simulink model "Sim7"  (R2014a)
settings: Solver=ode45  StartTime=0.0  StopTime=10.0  RelTol=1e-3
settings Model: Creator=OCAC  LastModifiedBy=OCAC

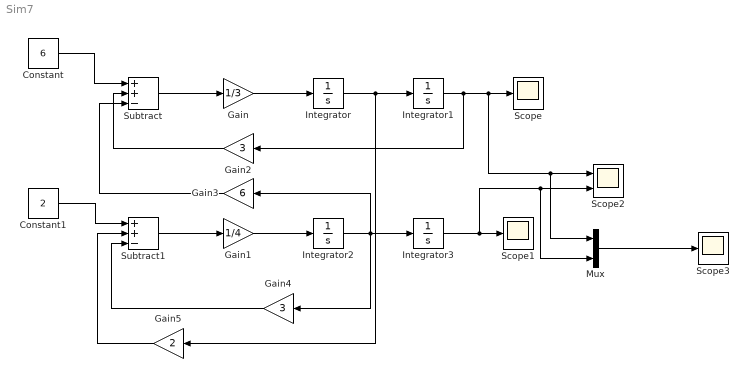
== system Sim7 ==
  Constant : Constant  Value=6
  Constant1 : Constant  Value=2
  Gain : Gain  Gain=1/3
  Gain1 : Gain  Gain=1/4
  Gain2 : Gain  Gain=3
  Gain3 : Gain  Gain=6
  Gain4 : Gain  Gain=3
  Gain5 : Gain  Gain=2
  Integrator{,1..3} (4 alike) : Integrator
  Mux : Mux  Inputs=2
  Scope : Scope
  Scope1 : Scope
  Scope2 : Scope  NumInputPorts=2
      settings: YMin=-5~-5  YMax=5~5  SaveName=ScopeData2
  Scope3 : Scope
      settings: SaveName=ScopeData3
  Subtract : Sum  Inputs=++-
  Subtract1 : Sum  Inputs=++-
  wires:
  Constant/1 -> Subtract/1
  Subtract/1 -> Gain/1
  Gain/1 -> Integrator/1
  Integrator/1 -> Gain5/1, Integrator1/1
  Constant1/1 -> Subtract1/1
  Subtract1/1 -> Gain1/1
  Gain1/1 -> Integrator2/1
  Integrator2/1 -> Gain4/1, Gain3/1, Integrator3/1
  Integrator1/1 -> Mux/1, Scope2/1, Scope/1, Gain2/1
  Gain2/1 -> Subtract/2
  Gain3/1 -> Subtract/3
  Gain4/1 -> Subtract1/3
  Gain5/1 -> Subtract1/2
  Integrator3/1 -> Mux/2, Scope2/2, Scope1/1
  Mux/1 -> Scope3/1
